simulink model "receive_test"  (R2021a)
settings: Solver=FixedStepAuto  StartTime=0.0  StopTime=10  RelTol=1e-3
libraries: instrumentseriallib x2
settings Model: Creator=surface  LastModifiedBy=surface
settings OptimizationCC: EnhancedBackFolding=on  PassReuseOutputArgsAs=Individual arguments  ZeroExternalMemoryAtStartup=off  ZeroInternalMemoryAtStartup=off  MaxStackSize=64  AccelVerboseBuild=on  OptimizeBlockOrder=speed  DifferentSizesBufferReuse=on  OptimizationCustomize=off  EfficientTunableParamExpr=on
settings DebuggingCC: ParameterTunabilityLossMsg=error
settings HardwareCC: ProdBitPerPointer=32  ProdBitPerSizeT=32  ProdBitPerPtrDiffT=32  ProdLargestAtomicFloat=None  ProdIntDivRoundTo=Undefined  ProdEndianess=Unspecified  ProdWordSize=32  ProdHWDeviceType=Generic->Unspecified (assume 32-bit Generic)
settings SFSimCC: SimDebugExecutionForCustomCode=on  MATLABDynamicMemAlloc=off  SimTargetLang=C++
settings RTWCC: SystemTargetFile=ert.tlc  HardwareBoard=Robot Operating System (ROS)  TLCOptions="-aInlineSetEventsForThisBaseRateFcn=TLC_FALSE -aSuppressMultiTaskScheduler=TLC_FALSE  -aRateBasedStepFcn=0"  TemplateMakefile=ert_default_tmf  Toolchain=Catkin  TargetLang=C++
settings CodeAppCC: ForceParamTrailComments=on  IgnoreCustomStorageClasses=off  OperatorAnnotations=on  SimulinkDataObjDesc=on  SFDataObjDesc=on  InsertBlockDesc=on

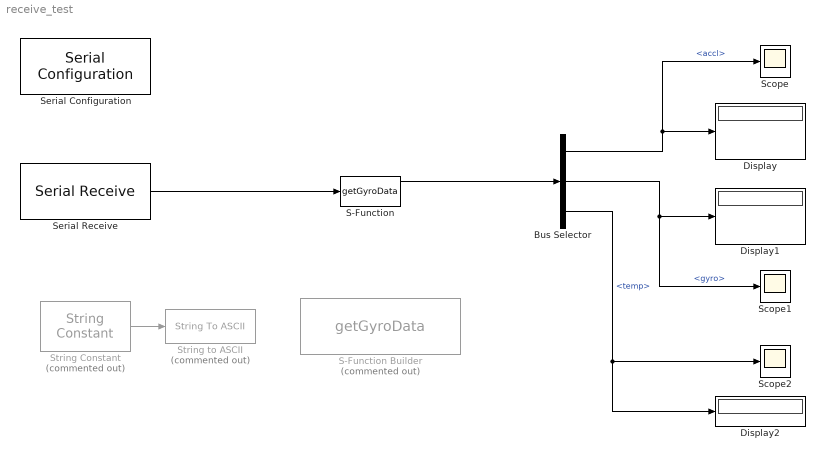
== system receive_test ==
  Bus Selector : BusSelector  OutputSignals=accl,gyro,temp
  Display : Display
      settings: Format=bank
  Display1 : Display
      settings: Format=bank
  Display2 : Display
      settings: Format=bank  Decimation=3
  S-Function : S-Function  FunctionName=getGyroData  SFunctionDeploymentMode=off  EnableBusSupport=off
  S-Function Builder : S-Function  Commented=on  FunctionName=getGyroData  SFunctionModules=getGyroData_wrapper  SFunctionDeploymentMode=off  EnableBusSupport=off  mask(S-Function Builder){}
      mask help: Simulink:masks:SFunctionBuilder_MD
      mask init:
      | val = [[.9  0.75 0.75 1 1 .9 .9 1]',[1 1 0.75 0.75 .9 .9 1 .9]'];try , sys = get_param(gcb,'SfunBuilderFcnName');if isempty(sys), sys = get_param(gcb,'FunctionName'); end,catch, sys = get_param(gcb,'FunctionName'); end
      settings: CopyFcn=set_param(gcbh,'LinkStatus','none')  OpenFcn=sfunctionwizard(gcbh)
      mask Display:
      | plot(val(:,1),val(:,2))
      | disp(sys)
      | port_label('input',1,'buffer')
      | port_label('output',1,'pData')
      | port_label('output',2,'str')
      | port_label('output',3,'len')
  Scope : Scope
  Scope1 : Scope
  Scope2 : Scope
  Serial Configuration : instrumentseriallib/Serial Configuration  Priority=-200000  Port=COM6  ComPort=COM6  BaudRate=115200  DataBits=8  Parity=none  StopBits=1  ByteOrder=little-endian  FlowControl=none  Timeout=10  SimulateUsing=Interpreted execution  BlockInModel=on
  Serial Receive : instrumentseriallib/Serial Receive  Priority=1  Port=COM6  ComPort=COM6  DataType=uint8  SaveDataType=uint8  ToggleHeader=off  Header=[91]  ToggleTerminator=off  Terminator=Custom terminator  CustomTerminator=[93]  ToggleDataSize=on  DataSize=128  EnableBlockingMode=on  ActionDataUnavailable=Output last received value  ActionWhenDataUnavailable=Output last received value  CustomValue=0  SampleTime=0.01  SimulateUsing=Interpreted execution  BlockInModel=on
  String Constant : StringConstant  Commented=on  String="\"1, Y = 122, Z=30\\nTemp=34.423]\\n[Accl X=101, Y = -111, Z=1023\\nGyro  X=-10231, Y = 1101, Z=0230\\nTemp=23.7893]\\n[Accl X=321, Y = -211, Z=-23\\nGyro  X=231, Y = 122, Z=30\\nTemp=33.643]\\n\""
  String to ASCII : StringToASCII  Commented=on  OutputVectorSize=128
  wires:
  S-Function/1 -> Bus Selector/1
  Bus Selector/1 -> Scope/1, Display/1  "<accl>"
  Bus Selector/2 -> Scope1/1, Display1/1  "<gyro>"
  String Constant/1 -> String to ASCII/1
  Bus Selector/3 -> Scope2/1, Display2/1  "<temp>"
  Serial Receive/1 -> S-Function/1
